simulink model "modelpid"  (Simulink 7.5)
settings: Solver=ode3  StartTime=0.0  StopTime=15.0  FixedStep=0.01  RelTol=1e-3
values from neighbouring files (symbols this model uses):
  kp = -5.5041440691    [konst_kp_ti_td.mat]
  td = 0.402735975267    [konst_kp_ti_td.mat]
  ti = 1.61094390107    [konst_kp_ti_td.mat]
libraries: simulink x1
settings Model: Creator=michal  LastModifiedBy=michal

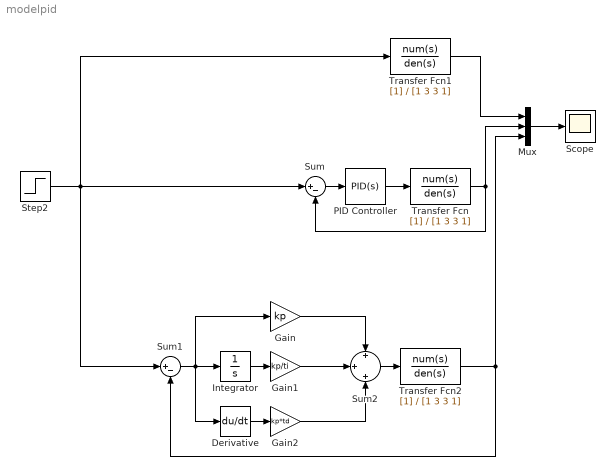
== system modelpid ==
  Derivative : Derivative
  Gain : Gain  Gain=kp  ParameterDataType=fixdt(1, 16)  ParameterScaling=2^0  OutDataType=fixdt(1, 16)  OutScaling=2^0
  Gain1 : Gain  Gain=kp/ti  ParameterDataType=fixdt(1, 16)  ParameterScaling=2^0  OutDataType=fixdt(1, 16)  OutScaling=2^0
  Gain2 : Gain  Gain=kp*td  ParameterDataType=fixdt(1, 16)  ParameterScaling=2^0  OutDataType=fixdt(1, 16)  OutScaling=2^0
  Integrator : Integrator
  Mux : Mux  Inputs=3
  PID Controller : simulink/Continuous/PID Controller  DialogController=pidpack.PIDConfig.pidDDGCreate  DialogControllerArgs=DataTag0  SystemSampleTime=-1  Controller=PID  TimeDomain=Continuous-time  SampleTime=1  IntegratorMethod=Forward Euler  FilterMethod=Forward Euler  Form=Parallel  P=kp  I=kp/ti  D=kp*td  N=100  InitialConditionSource=internal  InitialConditionForIntegrator=0  InitialConditionForFilter=0  ExternalReset=none  LimitOutput=off  UpperSaturationLimit=inf  LowerSaturationLimit=-inf  LinearizeAsGain=off  AntiWindupMode=none  Kb=1  TrackingMode=off  Kt=1  PParamMin=[]  PParamMax=[]  IParamMin=[]  IParamMax=[]  DParamMin=[]  DParamMax=[]  NParamMin=[]  NParamMax=[]  KbParamMin=[]  KbParamMax=[]  KtParamMin=[]  KtParamMax=[]  POutMin=[]  POutMax=[]  IOutMin=[]  IOutMax=[]  DOutMin=[]  DOutMax=[]  NOutMin=[]  NOutMax=[]  KbOutMin=[]  KbOutMax=[]  KtOutMin=[]  KtOutMax=[]  IntegratorOutMin=[]  IntegratorOutMax=[]  FilterOutMin=[]  FilterOutMax=[]  SumOutMin=[]  SumOutMax=[]  SumI1OutMin=[]  SumI1OutMax=[]  SumI2OutMin=[]  SumI2OutMax=[]  SumI3OutMin=[]  SumI3OutMax=[]  SumDOutMin=[]  SumDOutMax=[]  SaturationOutMin=[]  SaturationOutMax=[]  IntegratorContinuousStateAttributes=''  IntegratorStateMustResolveToSignalObject=off  IntegratorRTWStateStorageClass=Auto  FilterContinuousStateAttributes=''  FilterStateMustResolveToSignalObject=off  FilterRTWStateStorageClass=Auto
  Scope : Scope
      settings: DataFormat=Array
  Step2 : Step  Time=0  SampleTime=0
  Sum : Sum  Inputs=|+-  OutDataType=fixdt(1, 16)  OutScaling=2^0
  Sum1 : Sum  Inputs=|+-  OutDataType=fixdt(1, 16)  OutScaling=2^0
  Sum2 : Sum  Inputs=+|+|+  OutDataType=fixdt(1, 16)  OutScaling=2^0
  Transfer Fcn : TransferFcn  Denominator=[1 3 3 1]
  Transfer Fcn1 : TransferFcn  Denominator=[1 3 3 1]
  Transfer Fcn2 : TransferFcn  Denominator=[1 3 3 1]
  wires:
  Transfer Fcn/1 -> Mux/2, Sum/2
  Transfer Fcn1/1 -> Mux/1
  Mux/1 -> Scope/1
  Transfer Fcn2/1 -> Mux/3, Sum1/2
  Integrator/1 -> Gain1/1
  Derivative/1 -> Gain2/1
  Sum/1 -> PID Controller/1
  PID Controller/1 -> Transfer Fcn/1
  Gain/1 -> Sum2/1
  Gain1/1 -> Sum2/2
  Gain2/1 -> Sum2/3
  Sum2/1 -> Transfer Fcn2/1
  Sum1/1 -> Integrator/1, Gain/1, Derivative/1
  Step2/1 -> Sum1/1, Sum/1, Transfer Fcn1/1
